simulink model "cps_network_v2"  (R2012b)
settings: Solver=FixedStepDiscrete  StartTime=0.0  StopTime=10.0  RelTol=1e-3
settings Model: Creator=pmosterm  LastModifiedBy=pmosterm
settings SolverCC: EnableConcurrentExecution=on  ConcurrentTasks=on
settings DataIOCC: SignalLoggingSaveFormat=ModelDataLogs
settings OptimizationCC: InlineParams=on
settings DebuggingCC: UnderspecifiedInitializationDetection=Simplified  FcnCallInpInsideContextMsg=EnableAllAsWarning
settings ModelReferenceCC: ModelReferenceNumInstancesAllowed=Single
settings GRTTargetCC: CombineOutputUpdateFcns=off  GRTInterface=on

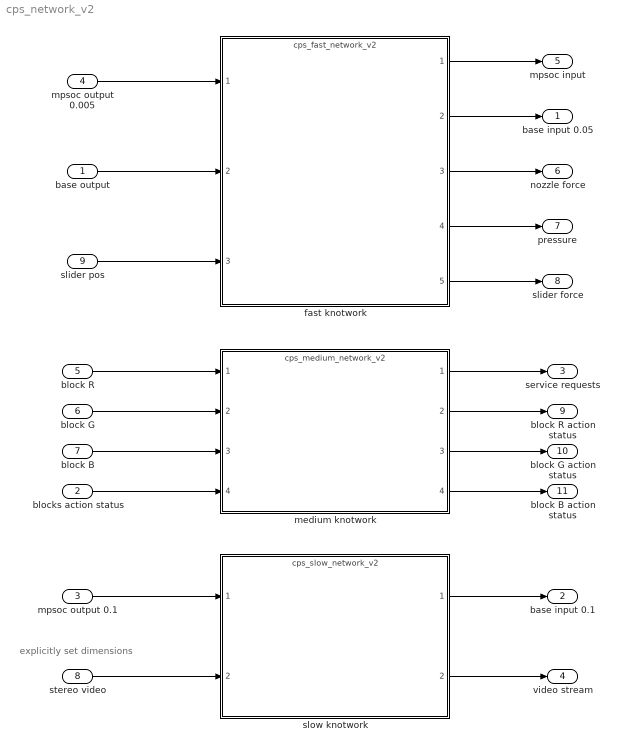
== system cps_network_v2 ==
  note: explicitly set dimensions
  base output : Inport  OutDataTypeStr=Bus: slBusBaseOps
  blocks action status : Inport  Port=2  SampleTime=0.05
  mpsoc output 0.1 : Inport  Port=3  OutDataTypeStr=Bus: slBusStereoOps
  mpsoc output 0.005 : Inport  Port=4  OutDataTypeStr=Bus: slBusNozzleControl
  block R : Inport  Port=5  OutDataTypeStr=Bus: slBusBlockOps  SampleTime=0.05  BusOutputAsStruct=on
  block G : Inport  Port=6  OutDataTypeStr=Bus: slBusBlockOps  SampleTime=0.05  BusOutputAsStruct=on
  block B : Inport  Port=7  OutDataTypeStr=Bus: slBusBlockOps  SampleTime=0.05  BusOutputAsStruct=on
  stereo video : Inport  Port=8  OutDataTypeStr=uint8  PortDimensions=[400 240 6]  SampleTime=0.1
  slider pos : Inport  Port=9
  fast knotwork : ModelReference  ModelNameDialog=cps_fast_network_v2  SimulationMode=Normal  ModelReferenceVersion=1.571  CopyOfModelName=cps_fast_network_v2  DefaultDataLogging=on
  medium knotwork : ModelReference  ModelNameDialog=cps_medium_network_v2  SimulationMode=Normal  ModelReferenceVersion=1.570  CopyOfModelName=cps_medium_network_v2  DefaultDataLogging=on
  slow knotwork : ModelReference  ModelNameDialog=cps_slow_network_v2  SimulationMode=Normal  ModelReferenceVersion=1.562  CopyOfModelName=cps_slow_network_v2  DefaultDataLogging=on
  base input 0.05 : Outport  OutDataTypeStr=Bus: slBusSliderStatus  SampleTime=0.005  BusOutputAsStruct=on
  base input 0.1 : Outport  Port=2  OutDataTypeStr=Bus: slBusStereoOps  SampleTime=0.1  BusOutputAsStruct=on
  service requests : Outport  Port=3  OutDataTypeStr=Bus: slBusBlockOps  PortDimensions=3  BusOutputAsStruct=on
  video stream : Outport  Port=4  SampleTime=0.1
  mpsoc input : Outport  Port=5  OutDataTypeStr=Bus: slBusSliderControlOps  BusOutputAsStruct=on
  nozzle force : Outport  Port=6
  pressure : Outport  Port=7
  slider force : Outport  Port=8
  block R action status : Outport  Port=9  BusOutputAsStruct=on
  block G action status : Outport  Port=10  BusOutputAsStruct=on
  block B action status : Outport  Port=11  BusOutputAsStruct=on
  wires:
  base output/1 -> fast knotwork/2
  mpsoc output 0.005/1 -> fast knotwork/1
  fast knotwork/4 -> pressure/1
  fast knotwork/5 -> slider force/1
  fast knotwork/3 -> nozzle force/1
  fast knotwork/2 -> base input 0.05/1
  slider pos/1 -> fast knotwork/3
  fast knotwork/1 -> mpsoc input/1
  mpsoc output 0.1/1 -> slow knotwork/1
  stereo video/1 -> slow knotwork/2
  block R/1 -> medium knotwork/1
  block G/1 -> medium knotwork/2
  blocks action status/1 -> medium knotwork/4
  medium knotwork/1 -> service requests/1
  medium knotwork/2 -> block R action status/1
  medium knotwork/3 -> block G action status/1
  slow knotwork/1 -> base input 0.1/1
  slow knotwork/2 -> video stream/1
  block B/1 -> medium knotwork/3
  medium knotwork/4 -> block B action status/1
